simulink library "speedgoatlib_IO511"  (R2012a)
settings: Solver=ode45  StartTime=0.0  StopTime=10.0  RelTol=1e-3
undefined symbols (not defined in the file): ATI, R5, RP, sg_IO511_intfilter_m, sg_IO511_rdhwfifo_m, sg_IO511_rdintvector_m, sg_IO511_setup_m, sg_IO511_txintenable_m, sg_IO511_wrhwfifo_m
libraries: speedgoatlib_IO511 x28, xpcseriallib x8, xpclib x2
Description:
  | 7.14.0.739 (R2012a)
settings Model: Creator=cschafft  LastModifiedBy=lab3

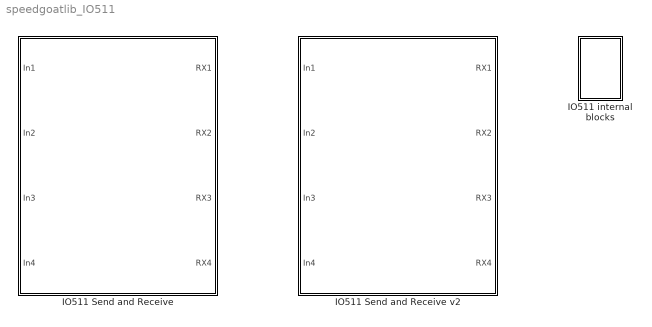
== system speedgoatlib_IO511 ==
  IO511 Send and Receive : Subsystem
      mask Display:
      | disp('IO511\nSpeedgoat\nSend\nReceive');
      | port_label('input', 1, 'Chan1 TX' );
      | port_label('input', 2, 'Chan2 TX' );
      | port_label('input', 3, 'Chan3 TX' );
      | port_label('input', 4, 'Chan4 TX' );
      | port_label('output', 1, 'Chan1 RX' );
      | port_label('output', 2, 'Chan2 RX' );
      | port_label('output', 3, 'Chan3 RX' );
      | port_label('output', 4, 'Chan4 RX' );
  IO511 Send and Receive v2 : Subsystem  mask(sendrecv_IO511){module_id=1, pci_slot=-1, channel_setup=1, channel1_mode=DTE, channel2_mode=DTE, channel3_mode=DCE, channel4_mode=DCE, channel1_freq=10e6, channel2_freq=10e6, channel3_freq=10e6, channel4_freq=10e6, channel1_fifo_threshold=2, channel2_fifo_threshold=2, channel3_fifo_threshold=2, channel4_fifo_threshold=2, channel1_data_size=2, channel2_data_size=2, channel3_data_size=2, channel4_data_size=2}
      mask prompts: module_id "Module identifier"; pci_slot "PCI slot (-1: autosearch)"; channel_setup "Channel setup"; channel1_mode "Mode"; channel2_mode "Mode"; channel3_mode "Mode"; channel4_mode "Mode"; channel1_freq "Frequency [Hz] (-1 if TX freq is cable sourced)"; channel2_freq "Frequency [Hz] (-1 if TX freq is cable sourced)"; channel3_freq "Frequency [Hz] (-1 if TX freq is cable sourced)"; channel4_freq "Frequency [Hz] (-1 if TX freq is cable sourced)"; channel1_fifo_threshold "RX FIFO almost full threshold"; channel2_fifo_threshold "RX FIFO almost full threshold"; channel3_fifo_threshold "RX FIFO almost full threshold"; channel4_fifo_threshold "RX FIFO almost full threshold"; channel1_data_size "Data size (count)"; channel2_data_size "Data size (count)"; channel3_data_size "Data size (count)"; channel4_data_size "Data size (count)"
      mask help: IO511 Send and Receive block
      mask init:
      | %set_param(gcb, 'LinkStatus', 'inactive');
      | mode_vect = nan;
      | freq_vect = nan; 
      | fifo_threshold_vect = nan;
      | sg_IO511_sendrecv_m(3);
      | sg_IO511_sendrecv_m(1, module_id, pci_slot, ...
      |                        mode_vect, channel1_mode, channel2_mode, channel3_mode, channel4_mode, ...
      |                        freq_vect, channel1_freq, channel2_freq, channel3_freq, channel4_freq, ...
      |                        fifo_threshold_vect, channel1_fifo_threshold, channel2_fifo_threshold, channel3_fifo_threshold, channel4_fifo_threshold, ...
      |                        channel1_data_size, channel2_data_size, channel3_data_size, channel4_data_size);
      mask Help: web(['C:\Users\lab3\Documents\MATLAB\trunk\thirdpartydrivers\sg_help\serial\dialog_fields_send_receive_io511.htm'],'-helpbrowser');
      mask StyleString: popup(1|2),edit,popup(1|2|3|4),popup(DTE|DCE),popup(DTE|DCE),popup(DTE|DCE),popup(DTE|DCE),edit,edit,edit,edit,edit,edit,edit,edit,edit,edit,edit,edit
      mask CallbackString: ||sg_IO511_sendrecv_m(2);||||||||||||||||
      mask Display:
      | disp('IO511\nSpeedgoat\nSend\nReceive');
      | port_label('input', 1, 'Chan1 TX' );
      | port_label('input', 2, 'Chan2 TX' );
      | port_label('input', 3, 'Chan3 TX' );
      | port_label('input', 4, 'Chan4 TX' );
      | port_label('output', 1, 'Chan1 RX' );
      | port_label('output', 2, 'Chan2 RX' );
      | port_label('output', 3, 'Chan3 RX' );
      | port_label('output', 4, 'Chan4 RX' );
  IO511 internal blocks : Subsystem

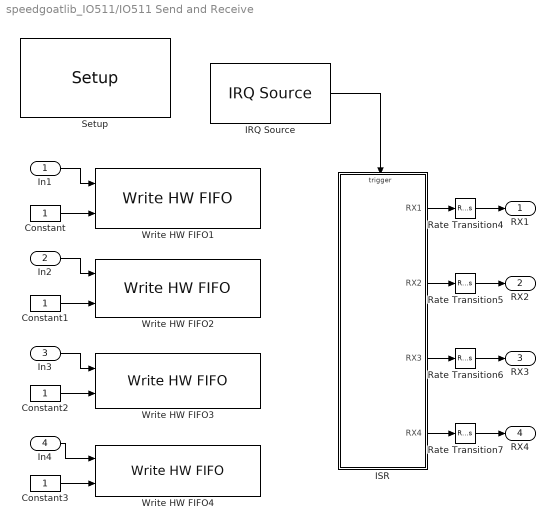
== system speedgoatlib_IO511/IO511 Send and Receive ==
  In1 : Inport
  In2 : Inport  Port=2
  In3 : Inport  Port=3
  In4 : Inport  Port=4
  Constant{,1..3} (4 alike) : Constant  OutDataTypeStr=Inherit: Inherit via back propagation
  IRQ Source : xpclib/Asynchronous Event/IRQ Source  irqNo=Auto (PCI only)  preempt=off  b_type=ATI-RP-R5  slot=-1
  ISR : Subsystem  TreatAsAtomicUnit=on
  Rate Transition{4..7} (4 alike) : RateTransition  Integrity=off  Deterministic=off
  Setup : speedgoatlib_IO511/IO511 internal blocks/Setup  id=1  chan=[1 2 3 4]  mode=[1 1 0 0]  freq=1e6  rxAlmost=[2 2 2 2]  pciSlot=-1
  Write HW FIFO1 : speedgoatlib_IO511/IO511 internal blocks/Write HW FIFO  id=1  chan=1  max=2  pciSlot=-1  ts=-1
  Write HW FIFO2 : speedgoatlib_IO511/IO511 internal blocks/Write HW FIFO  id=1  chan=2  max=2  pciSlot=-1  ts=-1
  Write HW FIFO3 : speedgoatlib_IO511/IO511 internal blocks/Write HW FIFO  id=1  chan=3  max=2  pciSlot=-1  ts=-1
  Write HW FIFO4 : speedgoatlib_IO511/IO511 internal blocks/Write HW FIFO  id=1  chan=4  max=2  pciSlot=-1  ts=-1
  RX1 : Outport
  RX2 : Outport  Port=2
  RX3 : Outport  Port=3
  RX4 : Outport  Port=4
  wires:
  In1/1 -> Write HW FIFO1/1
  In2/1 -> Write HW FIFO2/1
  In3/1 -> Write HW FIFO3/1
  In4/1 -> Write HW FIFO4/1
  Constant3/1 -> Write HW FIFO4/2
  Constant2/1 -> Write HW FIFO3/2
  Constant1/1 -> Write HW FIFO2/2
  Constant/1 -> Write HW FIFO1/2
  IRQ Source/1 -> ISR/Trigger
  Rate Transition4/1 -> RX1/1
  Rate Transition5/1 -> RX2/1
  Rate Transition6/1 -> RX3/1
  Rate Transition7/1 -> RX4/1
  ISR/1(RX1) -> Rate Transition4/1
  ISR/2(RX2) -> Rate Transition5/1
  ISR/3(RX3) -> Rate Transition6/1
  ISR/4(RX4) -> Rate Transition7/1

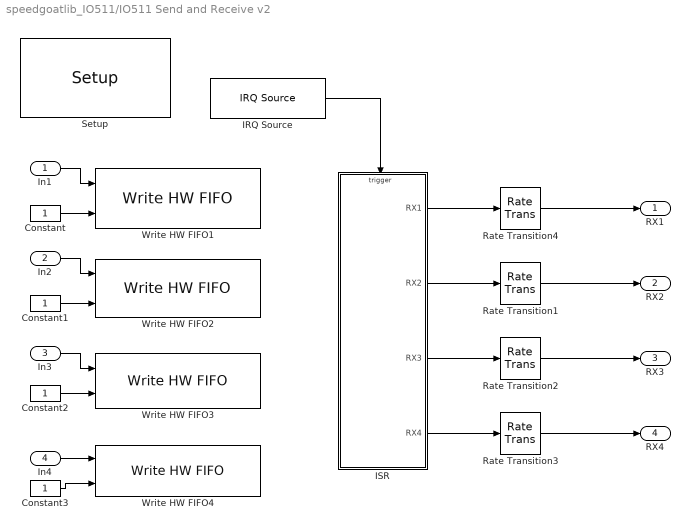
== system speedgoatlib_IO511/IO511 Send and Receive v2 ==
  In1 : Inport
  In2 : Inport  Port=2
  In3 : Inport  Port=3
  In4 : Inport  Port=4
  Constant{,1..3} (4 alike) : Constant  OutDataTypeStr=Inherit: Inherit via back propagation
  IRQ Source : xpclib/Asynchronous Event/IRQ Source  irqNo=Auto (PCI only)  preempt=off  b_type=ATI-RP-R5  slot=-1
  ISR : Subsystem  TreatAsAtomicUnit=on
  Rate Transition{1..4} (4 alike) : RateTransition  Integrity=off  Deterministic=off
  Setup : speedgoatlib_IO511/IO511 internal blocks/Setup  id=1  chan=[1 2 3 4]  mode=[0 0 1 1]  freq=[10000000 10000000 10000000 10000000]  rxAlmost=[2 2 2 2]  pciSlot=-1
  Write HW FIFO1 : speedgoatlib_IO511/IO511 internal blocks/Write HW FIFO  id=1  chan=1  max=2  pciSlot=-1  ts=-1
  Write HW FIFO2 : speedgoatlib_IO511/IO511 internal blocks/Write HW FIFO  id=1  chan=2  max=2  pciSlot=-1  ts=-1
  Write HW FIFO3 : speedgoatlib_IO511/IO511 internal blocks/Write HW FIFO  id=1  chan=3  max=2  pciSlot=-1  ts=-1
  Write HW FIFO4 : speedgoatlib_IO511/IO511 internal blocks/Write HW FIFO  id=1  chan=4  max=2  pciSlot=-1  ts=-1
  RX1 : Outport
  RX2 : Outport  Port=2
  RX3 : Outport  Port=3
  RX4 : Outport  Port=4
  wires:
  ISR/4(RX4) -> Rate Transition3/1
  ISR/3(RX3) -> Rate Transition2/1
  ISR/2(RX2) -> Rate Transition1/1
  ISR/1(RX1) -> Rate Transition4/1
  Rate Transition3/1 -> RX4/1
  Rate Transition2/1 -> RX3/1
  Rate Transition1/1 -> RX2/1
  Rate Transition4/1 -> RX1/1
  IRQ Source/1 -> ISR/Trigger
  Constant/1 -> Write HW FIFO1/2
  Constant1/1 -> Write HW FIFO2/2
  Constant2/1 -> Write HW FIFO3/2
  Constant3/1 -> Write HW FIFO4/2
  In4/1 -> Write HW FIFO4/1
  In3/1 -> Write HW FIFO3/1
  In2/1 -> Write HW FIFO2/1
  In1/1 -> Write HW FIFO1/1

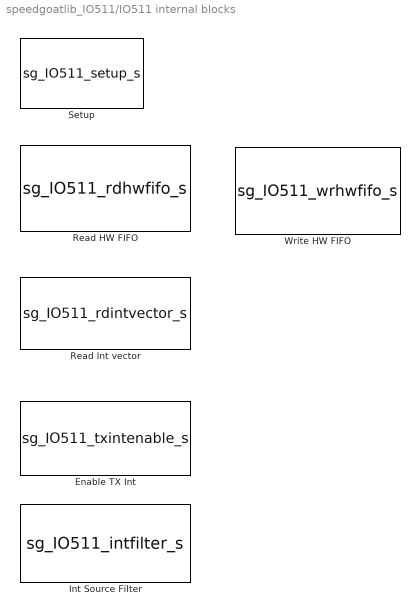
== system speedgoatlib_IO511/IO511 internal blocks ==
  Enable TX Int : S-Function  InitFcn=sg_IO511_txintenable_m(1);  FunctionName=sg_IO511_txintenable_s  Parameters=pciSlot, ts, chan  EnableBusSupport=off  mask(txintenable_IO511){id=1, chan=1, pciSlot=-1, ts=0.001}
      mask prompts: id "IO511 module identifier:"; chan "Channel:"; pciSlot "PCI slot (-1: autosearch):"; ts "Sample time:"
      mask help: Speedgoat driver block<br>IO511 - HDLC/SDLC enable TX interrupts<br><br>&copy; 2006 - 2012, Speedgoat GmbH, www.speedgoat.ch
      mask init:
      | sg_IO511_txintenable_m(3, id);
      mask Help: Documentation for this block is not available.
      mask StyleString: popup(1|2|3|4|5|6|7|8|9|10),edit,edit,edit
      mask Display: disp('Speedgoat\nIO511\nHDLC/SDLC enable TX int\nModule: 1');port_label('input', 1, 'DP');
  Int Source Filter : S-Function  InitFcn=sg_IO511_intfilter_m(1);  FunctionName=sg_IO511_intfilter_s  Parameters=pciSlot,ts,dir,chan,width  EnableBusSupport=off  mask(intfilter_IO511){id=1, chan=1, dir=1, width=1, ts=-1, pciSlot=-1}
      mask prompts: id "IO511 module identifier:"; chan "Channel:"; dir "Direction (TX: 0, RX: 1, USC: 2):"; ts "Sample time:"; pciSlot "PCI slot (-1: autosearch):"
      mask help: Speedgoat driver block<br>IO511 - HDLC/SDLC interrupts source filter<br><br>&copy; 2006 - 2012, Speedgoat GmbH, www.speedgoat.ch
      mask init:
      | sg_IO511_intfilter_m(3, id);
      mask Help: Documentation for this block is not available.
      mask StyleString: popup(1|2|3|4|5|6|7|8|9|10),edit,edit,edit,edit,edit
      mask Display: disp('Speedgoat\nIO511\nHDLC/SDLC int filter\nModule: 1');port_label('input', 1, 'S');port_label('output', 1, 'E');
  Read HW FIFO : S-Function  InitFcn=sg_IO511_rdhwfifo_m(1);  FunctionName=sg_IO511_rdhwfifo_s  Parameters=pciSlot, ts, chan, fifoSize  EnableBusSupport=off  mask(rdhwfifo_IO511){id=1, chan=1, fifoSize=1, pciSlot=-1, ts=-1}
      mask prompts: id "IO511 module identifier:"; chan "Channel:"; fifoSize "FIFO size to read:"; pciSlot "PCI slot (-1: autosearch):"; ts "Sample time:"
      mask help: Speedgoat driver block<br>IO511 - HDLC/SDLC read HW FIFO<br><br>&copy; 2006 - 2012, Speedgoat GmbH, www.speedgoat.ch
      mask init:
      | sg_IO511_rdhwfifo_m(3, id);
      mask Help: Documentation for this block is not available.
      mask StyleString: popup(1|2|3|4|5|6|7|8|9|10),edit,edit,edit,edit
      mask Display: disp('Speedgoat\nIO511\nHDLC/SDLC read HW FIFO\nModule: 1');port_label('input', 1, 'E');port_label('output', 1, 'D');
  Read Int vector : S-Function  InitFcn=sg_IO511_rdintvector_m(1);  FunctionName=sg_IO511_rdintvector_s  Parameters=pciSlot,ts  EnableBusSupport=off  mask(rdintvector_IO511){id=1, ts=-1, pciSlot=-1}
      mask prompts: id "IO511 module identifier:"; ts "Sample time:"; pciSlot "PCI slot (-1: autosearch):"
      mask help: Speedgoat driver block<br>IO511 - HDLC/SDLC read interrupt vector<br><br>&copy; 2006 - 2012, Speedgoat GmbH, www.speedgoat.ch
      mask init:
      | sg_IO511_rdintvector_m(3, id);
      mask Help: Documentation for this block is not available.
      mask StyleString: popup(1|2|3|4|5|6|7|8|9|10),edit,edit
      mask Display: disp('Speedgoat\nIO511\nHDLC/SDLC read int\nModule: 1');port_label('output', 1, 'S');
  Setup : S-Function  InitFcn=sg_IO511_setup_m(1);  FunctionName=sg_IO511_setup_s  Parameters=pciSlot, chan, mode, freq, rxAlmost  EnableBusSupport=off  mask(setup_IO511){id=1, chan=[1 2 3 4], mode=[0 0 1 1], freq=[8e6 8e6 8e6 8e6], rxAlmost=[2 2 2 2], pciSlot=-1}
      mask prompts: id "IO511 module identifier:"; chan "Channels:"; mode "Mode (0: DTE, 1: DCE):"; freq "Frequency [Hz] (-1: if TX freq is cable sourced):"; rxAlmost "RX FIFO almost full threshold:"; pciSlot "PCI slot (-1: autosearch):"
      mask help: Speedgoat driver block<br>IO511 - Setup<br><br>&copy; 2006 - 2012, Speedgoat GmbH, www.speedgoat.ch
      mask init:
      | sg_IO511_setup_m(3, id, pciSlot);
      | iocr = 0;
      mask Help: Documentation for this block is not available.
      mask StyleString: popup(1|2|3|4|5|6|7|8|9|10),edit,edit,edit,edit,edit
      mask Display: disp('Speedgoat\nIO511\nSetup\nModule: 1');
  Write HW FIFO : S-Function  InitFcn=sg_IO511_wrhwfifo_m(1);  FunctionName=sg_IO511_wrhwfifo_s  Parameters=pciSlot, ts, chan, max  EnableBusSupport=off  mask(wrhwfifo_IO511){id=1, chan=1, max=64, pciSlot=-1, ts=-1}
      mask prompts: id "IO511 module identifier:"; chan "Channel:"; max "Maximum data to be written to software FIFO:"; pciSlot "PCI slot (-1: autosearch):"; ts "Sample time:"
      mask help: Speedgoat driver block<br>IO511 - HDLC/SDLC write HW FIFO<br><br>&copy; 2006 - 2012, Speedgoat GmbH, www.speedgoat.ch
      mask init:
      | sg_IO511_wrhwfifo_m(3, id);
      mask Help: Documentation for this block is not available.
      mask StyleString: popup(1|2|3|4|5|6|7|8|9|10),edit,edit,edit,edit
      mask Display: disp('Speedgoat\nIO511\nHDLC/SDLC write HW FIFO\nModule: 1');port_label('input', 1, 'D');port_label('input', 2, 'E');

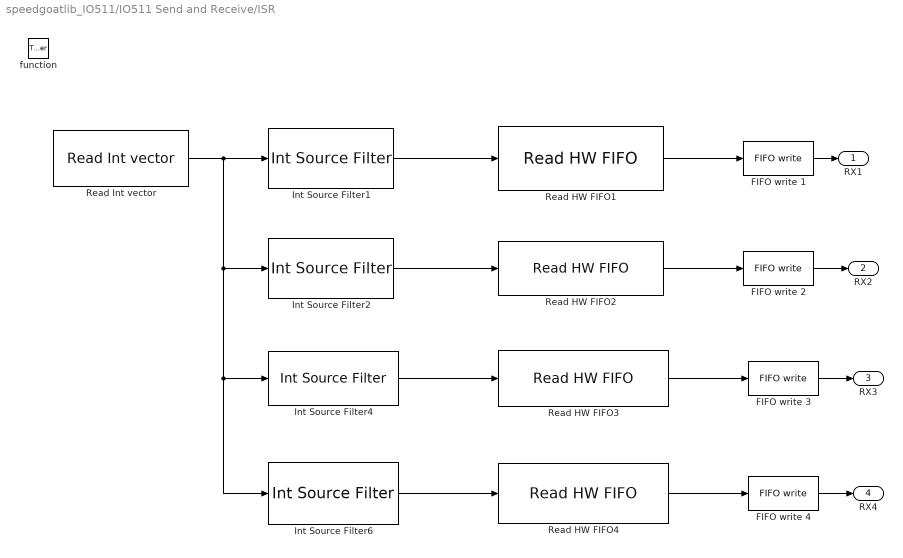
== system speedgoatlib_IO511/IO511 Send and Receive/ISR ==
  function : TriggerPort  TriggerType=function-call
  FIFO write 1 : xpcseriallib/FIFO write   size=1024  inputtype=count+16 bit uint  present=off  sampletime=-1  id=RCV channel 1
  FIFO write 2 : xpcseriallib/FIFO write   size=1024  inputtype=count+16 bit uint  present=off  sampletime=-1  id=RCV channel 2
  FIFO write 3 : xpcseriallib/FIFO write   size=1024  inputtype=count+16 bit uint  present=off  sampletime=-1  id=RCV channel 3
  FIFO write 4 : xpcseriallib/FIFO write   size=1024  inputtype=count+16 bit uint  present=off  sampletime=-1  id=RCV channel 4
  Int Source Filter1 : speedgoatlib_IO511/IO511 internal blocks/Int Source Filter  id=1  chan=1  dir=1  width=2  ts=-1  pciSlot=-1
  Int Source Filter2 : speedgoatlib_IO511/IO511 internal blocks/Int Source Filter  id=1  chan=2  dir=1  width=2  ts=-1  pciSlot=-1
  Int Source Filter4 : speedgoatlib_IO511/IO511 internal blocks/Int Source Filter  id=1  chan=3  dir=1  width=2  ts=-1  pciSlot=-1
  Int Source Filter6 : speedgoatlib_IO511/IO511 internal blocks/Int Source Filter  id=1  chan=4  dir=1  width=2  ts=-1  pciSlot=-1
  Read HW FIFO1 : speedgoatlib_IO511/IO511 internal blocks/Read HW FIFO  id=1  chan=1  fifoSize=64  pciSlot=-1  ts=-1
  Read HW FIFO2 : speedgoatlib_IO511/IO511 internal blocks/Read HW FIFO  id=1  chan=2  fifoSize=64  pciSlot=-1  ts=-1
  Read HW FIFO3 : speedgoatlib_IO511/IO511 internal blocks/Read HW FIFO  id=1  chan=3  fifoSize=64  pciSlot=-1  ts=-1
  Read HW FIFO4 : speedgoatlib_IO511/IO511 internal blocks/Read HW FIFO  id=1  chan=4  fifoSize=64  pciSlot=-1  ts=-1
  Read Int vector : speedgoatlib_IO511/IO511 internal blocks/Read Int vector  id=1  ts=-1  pciSlot=-1
  RX1 : Outport
  RX2 : Outport  Port=2
  RX3 : Outport  Port=3
  RX4 : Outport  Port=4
  wires:
  Read HW FIFO1/1 -> FIFO write 1/1
  FIFO write 1/1 -> RX1/1
  Int Source Filter1/1 -> Read HW FIFO1/1
  Read Int vector/1 -> Int Source Filter6/1, Int Source Filter4/1, Int Source Filter2/1, Int Source Filter1/1
  Int Source Filter6/1 -> Read HW FIFO4/1
  Int Source Filter4/1 -> Read HW FIFO3/1
  Read HW FIFO2/1 -> FIFO write 2/1
  FIFO write 2/1 -> RX2/1
  Read HW FIFO3/1 -> FIFO write 3/1
  FIFO write 3/1 -> RX3/1
  Read HW FIFO4/1 -> FIFO write 4/1
  FIFO write 4/1 -> RX4/1
  Int Source Filter2/1 -> Read HW FIFO2/1

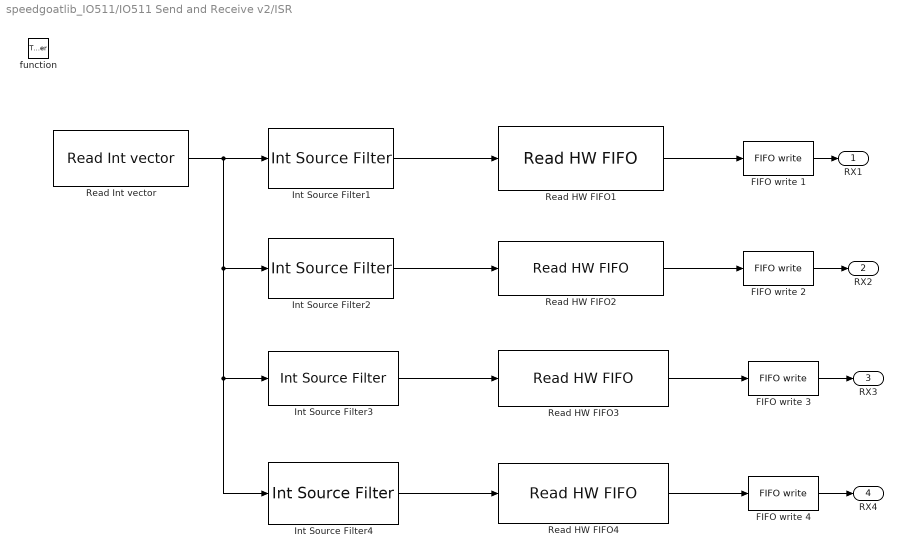
== system speedgoatlib_IO511/IO511 Send and Receive v2/ISR ==
  function : TriggerPort  TriggerType=function-call
  FIFO write 1 : xpcseriallib/FIFO write   size=1024  inputtype=count+16 bit uint  present=off  sampletime=-1  id=IO511 RCV channel 1
  FIFO write 2 : xpcseriallib/FIFO write   size=1024  inputtype=count+16 bit uint  present=off  sampletime=-1  id=IO511 RCV channel 2
  FIFO write 3 : xpcseriallib/FIFO write   size=1024  inputtype=count+16 bit uint  present=off  sampletime=-1  id=IO511 RCV channel 3
  FIFO write 4 : xpcseriallib/FIFO write   size=1024  inputtype=count+16 bit uint  present=off  sampletime=-1  id=IO511 RCV channel 4
  Int Source Filter1 : speedgoatlib_IO511/IO511 internal blocks/Int Source Filter  id=1  chan=1  dir=1  width=2  ts=-1  pciSlot=-1
  Int Source Filter2 : speedgoatlib_IO511/IO511 internal blocks/Int Source Filter  id=1  chan=2  dir=1  width=2  ts=-1  pciSlot=-1
  Int Source Filter3 : speedgoatlib_IO511/IO511 internal blocks/Int Source Filter  id=1  chan=3  dir=1  width=2  ts=-1  pciSlot=-1
  Int Source Filter4 : speedgoatlib_IO511/IO511 internal blocks/Int Source Filter  id=1  chan=4  dir=1  width=2  ts=-1  pciSlot=-1
  Read HW FIFO1 : speedgoatlib_IO511/IO511 internal blocks/Read HW FIFO  id=1  chan=1  fifoSize=1024  pciSlot=-1  ts=-1
  Read HW FIFO2 : speedgoatlib_IO511/IO511 internal blocks/Read HW FIFO  id=1  chan=2  fifoSize=1024  pciSlot=-1  ts=-1
  Read HW FIFO3 : speedgoatlib_IO511/IO511 internal blocks/Read HW FIFO  id=1  chan=3  fifoSize=1024  pciSlot=-1  ts=-1
  Read HW FIFO4 : speedgoatlib_IO511/IO511 internal blocks/Read HW FIFO  id=1  chan=4  fifoSize=1024  pciSlot=-1  ts=-1
  Read Int vector : speedgoatlib_IO511/IO511 internal blocks/Read Int vector  id=1  ts=-1  pciSlot=-1
  RX1 : Outport
  RX2 : Outport  Port=2
  RX3 : Outport  Port=3
  RX4 : Outport  Port=4
  wires:
  Int Source Filter2/1 -> Read HW FIFO2/1
  FIFO write 4/1 -> RX4/1
  Read HW FIFO4/1 -> FIFO write 4/1
  FIFO write 3/1 -> RX3/1
  Read HW FIFO3/1 -> FIFO write 3/1
  FIFO write 2/1 -> RX2/1
  Read HW FIFO2/1 -> FIFO write 2/1
  Int Source Filter3/1 -> Read HW FIFO3/1
  Int Source Filter4/1 -> Read HW FIFO4/1
  Read Int vector/1 -> Int Source Filter1/1, Int Source Filter2/1, Int Source Filter3/1, Int Source Filter4/1
  Int Source Filter1/1 -> Read HW FIFO1/1
  FIFO write 1/1 -> RX1/1
  Read HW FIFO1/1 -> FIFO write 1/1
